simulink model "SymmetricalBridgeConverter"  (R2013a)
settings: Solver=ode45  StartTime=0.0  StopTime=10.0  RelTol=1e-3
libraries: powerlib x12
settings Model: Creator=avirup  LastModifiedBy=avirup

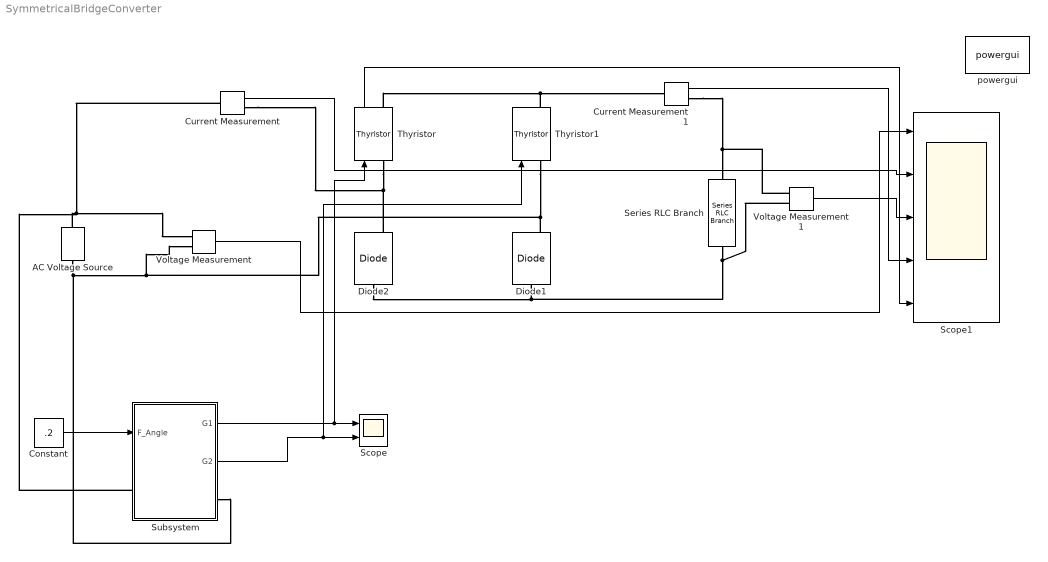
== system SymmetricalBridgeConverter ==
  AC Voltage Source : powerlib/Electrical Sources/AC Voltage Source  Amplitude=100  Phase=0  Frequency=60  SampleTime=0  Measurements=None
  Constant : Constant  Value=.2
  Current Measurement : powerlib/Measurements/Current Measurement  PhasorSimulation=off  OutputType=Complex  PSBequivalent=0
  Current Measurement1 : powerlib/Measurements/Current Measurement  PhasorSimulation=off  OutputType=Complex  PSBequivalent=0
  Diode1 : powerlib/Power Electronics/Diode  Ron=0.001  Lon=0  Vf=0.8  IC=0  UseSnubber=off  Rs=500  Cs=250e-9  Measurements=on
  Diode2 : powerlib/Power Electronics/Diode  Ron=0.001  Lon=0  Vf=0.8  IC=0  UseSnubber=off  Rs=500  Cs=250e-9  Measurements=on
  Scope : Scope  NumInputPorts=2
      settings: YMin=-5~-5  YMax=5~5  SaveName=ScopeData3
  Scope1 : Scope  NumInputPorts=5
      settings: YMin=-5~-5~-5~-5~-5  YMax=5~5~5~5~5  SaveName=ScopeData4
  Series RLC Branch : powerlib/Elements/Series RLC Branch  LConnTagsString=__new0  RConnTagsString=__new0  BranchType=RL  Resistance=1  Inductance=1e-3  SetiL0=off  InitialCurrent=0  Capacitance=1e-6  Setx0=off  InitialVoltage=0  Measurements=None
  Subsystem : Subsystem
  Thyristor : powerlib/Power Electronics/Thyristor  Ron=0.001  Lon=0  Vf=0.8  IC=0  Rs=500  Cs=250e-9  Measurements=on
  Thyristor1 : powerlib/Power Electronics/Thyristor  Ron=0.001  Lon=0  Vf=0.8  IC=0  Rs=500  Cs=250e-9  Measurements=on
  Voltage Measurement : powerlib/Measurements/Voltage Measurement  PhasorSimulation=off  OutputType=Complex  PSBequivalent=0
  Voltage Measurement1 : powerlib/Measurements/Voltage Measurement  PhasorSimulation=off  OutputType=Complex  PSBequivalent=0
  powergui : powerlib/powergui  Priority=1  SimulationMode=Continuous  SolverType=Tustin  SampleTime=50e-6  frequency=60  SPID=off  DisableSnubberDevices=off  DisableRonSwitches=off  DisableVfSwitches=off  SwTol=0  Interpol=off  DisplayEquations=off  frequencyindice=60  Pbase=100e6  ErrMax=1e-4  Iterations=50  UnitsV=kV  UnitsW=MW  FunctionMessages=off  echomessages=off  HookPort=off  EnableUseOfTLC=off  x0status=blocks  RestoreLinks=warning  ResistiveCurrentMeasurement=off  Frange=[0:2:500]  Ylog=off  Xlog=on  ShowGrid=off  save=off  variable=ZData  ZoomFFT=off  StartTime=0.0  cycles=1  DisplayStyle=1  fundamental=60  FreqAxis=off  MaxFrequency=1000  frequencyindicesteady=1  RmsSteady=1  display=off  Ts=0  methode=off
  wires:
  Constant/1 -> Subsystem/1(F_Angle)
  Subsystem/1(G1) -> Thyristor/1, Scope/1
  Subsystem/2(G2) -> Thyristor1/1, Scope/2
  Voltage Measurement/1 -> Scope1/1
  Current Measurement/1 -> Scope1/2
  Voltage Measurement1/1 -> Scope1/3
  Current Measurement1/1 -> Scope1/4
  Thyristor/1 -> Scope1/5
  connections:
  AC Voltage Source/RConn1 -- Current Measurement/LConn1 -- Subsystem/LConn1 -- Voltage Measurement/LConn1
  AC Voltage Source/LConn1 -- Subsystem/RConn1 -- Thyristor1/LConn1 -- Diode1/RConn1 -- Voltage Measurement/LConn2
  Thyristor/LConn1 -- Diode2/RConn1 -- Current Measurement/RConn1
  Thyristor/RConn1 -- Thyristor1/RConn1 -- Current Measurement1/LConn1
  Series RLC Branch/RConn1 -- Voltage Measurement1/LConn2 -- Diode2/LConn1 -- Diode1/LConn1
  Current Measurement1/RConn1 -- Voltage Measurement1/LConn1 -- Series RLC Branch/LConn1

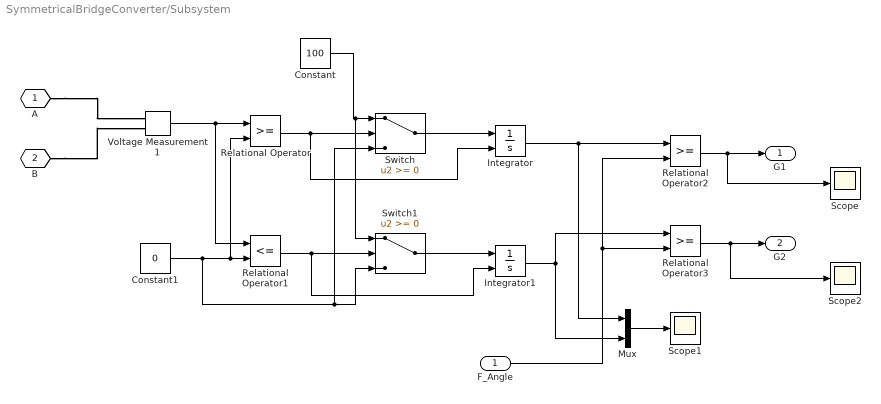
== system SymmetricalBridgeConverter/Subsystem ==
  F_Angle : Inport
  Constant : Constant  Value=100
  Constant1 : Constant  Value=0
  Integrator : Integrator  ExternalReset=falling
  Integrator1 : Integrator  ExternalReset=falling
  Mux : Mux  Inputs=2
  Relational Operator : RelationalOperator  OutDataTypeStr=boolean
  Relational Operator1 : RelationalOperator  Operator=<=  OutDataTypeStr=boolean
  Relational Operator2 : RelationalOperator  OutDataTypeStr=boolean
  Relational Operator3 : RelationalOperator  OutDataTypeStr=boolean
  Scope : Scope
  Scope1 : Scope
  Scope2 : Scope
      settings: SaveName=ScopeData2
  Switch : Switch
  Switch1 : Switch
  Voltage Measurement1 : powerlib/Measurements/Voltage Measurement  PhasorSimulation=off  OutputType=Complex  PSBequivalent=0
  A : PMIOPort  Tag=PMCPort  Port=1  Side=Left
  B : PMIOPort  Tag=PMCPort  Port=2  Side=Right
  G1 : Outport
  G2 : Outport  Port=2
  wires:
  Mux/1 -> Scope1/1
  Relational Operator2/1 -> G1/1, Scope/1
  Switch1/1 -> Integrator1/1
  Switch/1 -> Integrator/1
  Relational Operator/1 -> Integrator/2, Switch/2
  Relational Operator1/1 -> Integrator1/2, Switch1/2
  Constant1/1 -> Switch/3, Switch1/3, Relational Operator/2, Relational Operator1/2
  Constant/1 -> Switch1/1, Switch/1
  Voltage Measurement1/1 -> Relational Operator1/1, Relational Operator/1
  Integrator/1 -> Relational Operator2/1, Mux/1
  Integrator1/1 -> Relational Operator3/1, Mux/2
  F_Angle/1 -> Relational Operator2/2, Relational Operator3/2
  Relational Operator3/1 -> G2/1, Scope2/1
  connections:
  B/RConn1 -- Voltage Measurement1/LConn2
  A/RConn1 -- Voltage Measurement1/LConn1
